simulink model "pendulum_cart"  (R2020a)
settings: Solver=VariableStepAuto  StartTime=0.0  StopTime=15.0  MaxStep=0.01  RelTol=1e-3
libraries: simulink x1, simulink_extras x1
settings Model: Creator=kiril_000  LastModifiedBy=kiril_000

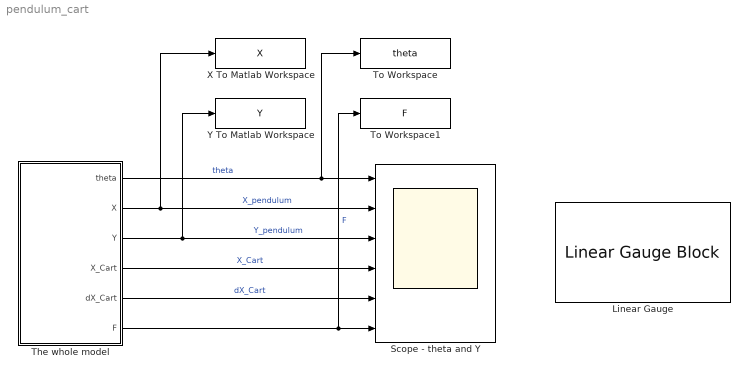
== system pendulum_cart ==
  Linear Gauge : LinearGaugeBlock  ScaleMin=-90  ScaleMax=90
  Scope - theta and Y : Scope  NumInputPorts=6
  The whole model : Subsystem  mask{m=1, M_Cart=3, l=1}
      mask prompts: m "Масса маятника"; M_Cart "Масса тележки"; l "Длина"
  To Workspace : ToWorkspace  VariableName=theta  SaveFormat=Timeseries  SampleTime=-1
  To Workspace1 : ToWorkspace  VariableName=F  SaveFormat=Timeseries  SampleTime=-1
  X To Matlab Workspace : ToWorkspace  VariableName=X  SampleTime=-1
      settings: Save2DSignal=2-D array (concatenate along first dimension)
  Y To Matlab Workspace : ToWorkspace  VariableName=Y  SampleTime=-1
      settings: Save2DSignal=2-D array (concatenate along first dimension)
  wires:
  The whole model/2(X) -> X To Matlab Workspace/1, Scope - theta and Y/2  "X_pendulum"
  The whole model/3(Y) -> Y To Matlab Workspace/1, Scope - theta and Y/3  "Y_pendulum"
  The whole model/1(theta) -> To Workspace/1, Scope - theta and Y/1  "theta"
  The whole model/4(X_Cart) -> Scope - theta and Y/4  "X_Cart"
  The whole model/5(dX_Cart) -> Scope - theta and Y/5  "dX_Cart"
  The whole model/6(F) -> To Workspace1/1, Scope - theta and Y/6  "F"

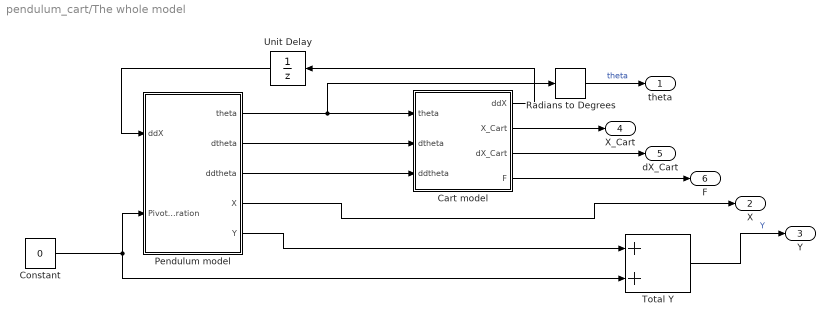
== system pendulum_cart/The whole model ==
  Cart model : Subsystem
  Constant : Constant  Value=0
  Pendulum model : Subsystem  mask{m=1, l=1, g=9.8, b=0.5}
      mask prompts: m "Масса"; l "Длина"; g "Ускорение свободного падения"; b "Коэффициент вязкости"
      mask init:
      | I = m * l^2;
  Radians to Degrees : simulink_extras/Transformations/Radians to Degrees
  Total Y : Sum
  Unit Delay : UnitDelay  SampleTime=-1  HasFrameUpgradeWarning=on
  theta : Outport
  X : Outport  Port=2
  Y : Outport  Port=3
  X_Cart : Outport  Port=4
  dX_Cart : Outport  Port=5
  F : Outport  Port=6
  wires:
  Radians to Degrees/1 -> theta/1  "theta"
  Cart model/1(ddX) -> Unit Delay/1
  Pendulum model/3(ddtheta) -> Cart model/3(ddtheta)
  Pendulum model/1(theta) -> Radians to Degrees/1, Cart model/1(theta)
  Pendulum model/5(Y) -> Total Y/1
  Pendulum model/4(X) -> X/1
  Pendulum model/2(dtheta) -> Cart model/2(dtheta)
  Total Y/1 -> Y/1  "Y"
  Constant/1 -> Total Y/2, Pendulum model/2(Pivot Acceleration)
  Cart model/2(X_Cart) -> X_Cart/1
  Cart model/3(dX_Cart) -> dX_Cart/1
  Cart model/4(F) -> F/1
  Unit Delay/1 -> Pendulum model/1(ddX)

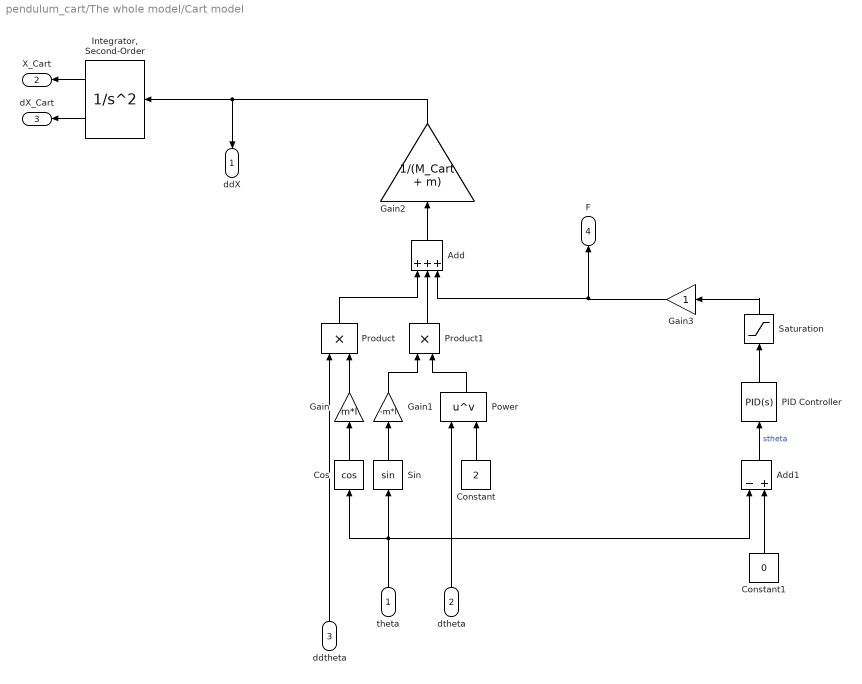
== system pendulum_cart/The whole model/Cart model ==
  theta : Inport
  dtheta : Inport  Port=2
  ddtheta : Inport  Port=3
  Add : Sum  Inputs=+++
  Add1 : Sum  Inputs=-+
  Constant : Constant  Value=2
  Constant1 : Constant  Value=0
  Cos : Trigonometry  Operator=cos
  Gain : Gain  Gain=m*l
  Gain1 : Gain  Gain=-m*l
  Gain2 : Gain  Gain=1/(M_Cart + m)
  Gain3 : Gain
  "Integrator, Second-Order" : SecondOrderIntegrator
  PID Controller : simulink/Continuous/PID Controller  Controller=PID  Form=Parallel  TimeDomain=Continuous-time  UseExternalTs=off  SampleTime=-1  IntegratorMethod=Forward Euler  FilterMethod=Forward Euler  ControllerParametersSource=internal  P=48  I=0  D=3  UseFilter=on  N=100  TunerSelectOption=Transfer Function Based (PID Tuner App)  InitialConditionSource=internal  InitialConditionForIntegrator=0  InitialConditionForFilter=0  DifferentiatorICPrevScaledInput=0  ExternalReset=none  TrackingMode=off  Kt=1  LimitOutput=off  UpperSaturationLimit=inf  LowerSaturationLimit=-inf  LinearizeAsGain=on  AntiWindupMode=none  Kb=1  POutMin=[]  POutMax=[]  IOutMin=[]  IOutMax=[]  DOutMin=[]  DOutMax=[]  NOutMin=[]  NOutMax=[]  SumOutMin=[]  SumOutMax=[]  SaturationOutMin=[]  SaturationOutMax=[]  PParamMin=[]  PParamMax=[]  IParamMin=[]  IParamMax=[]  DParamMin=[]  DParamMax=[]  NParamMin=[]  NParamMax=[]  KbParamMin=[]  KbParamMax=[]  KtParamMin=[]  KtParamMax=[]  KbOutMin=[]  KbOutMax=[]  KtOutMin=[]  KtOutMax=[]  IntegratorOutMin=[]  IntegratorOutMax=[]  FilterOutMin=[]  FilterOutMax=[]  SumI1OutMin=[]  SumI1OutMax=[]  SumI2OutMin=[]  SumI2OutMax=[]  SumI3OutMin=[]  SumI3OutMax=[]  SumI4OutMin=[]  SumI4OutMax=[]  SumDOutMin=[]  SumDOutMax=[]  DifferentiatorOutMin=[]  DifferentiatorOutMax=[]  FilterDiffOutCoefMin=[]  FilterDiffOutCoefMax=[]  ReciprocalOutMin=[]  ReciprocalOutMax=[]  SumDenOutMin=[]  SumDenOutMax=[]  SumNumOutMin=[]  SumNumOutMax=[]  DivideOutMin=[]  DivideOutMax=[]  UdiffTsProdOutMin=[]  UdiffTsProdOutMax=[]  NTsProdOutMin=[]  NTsProdOutMax=[]  UintegralTsProdOutMin=[]  UintegralTsProdOutMax=[]  UngainTsProdOutMin=[]  UngainTsProdOutMax=[]  IntegratorContinuousStateAttributes=''  IntegratorStateMustResolveToSignalObject=off  IntegratorRTWStateStorageClass=Auto  FilterContinuousStateAttributes=''  FilterStateMustResolveToSignalObject=off  FilterRTWStateStorageClass=Auto  ParallelPVariant=InternalParameters  IdealPVariant=Disabled  IVariant=InternalParameters  DVariant=InternalParameters  IntegratorVariant=Continuous  SatVariant=Disabled  AWVariant=Passthrough  PCopyVariant=Disabled  TRVariant=Disabled  FdbkBlocksVariant=Forward  IdealPFdbkVariant=Disabled  SatFdbkVariant=Disabled  DerivativeFilterVariant=ContFilter  NVariant=InternalParameters  NCopyVariant=Disabled  FilterICVariant=InternalICsFilter  IntegratorICVariant=InternalICs  ExternalResetVariant=Disabled  TRSumVariant=Passthrough  SumFdbkVariant=Disabled  SumVariant=Sum_PID  TsampFilterVariant=InternalTs  TsampNgainVariant=Passthrough  TsampIntegralVariant=Passthrough
  Power : Math  Operator=pow  SaturateOnIntegerOverflow=on
  Product : Product
  Product1 : Product
  Saturation : Saturate  UpperLimit=5  LowerLimit=-5
  Sin : Trigonometry
  ddX : Outport
  X_Cart : Outport  Port=2
  dX_Cart : Outport  Port=3
  F : Outport  Port=4
  wires:
  Sin/1 -> Gain1/1
  Cos/1 -> Gain/1
  Product1/1 -> Add/2
  Power/1 -> Product1/2
  Gain1/1 -> Product1/1
  Add/1 -> Gain2/1
  Constant/1 -> Power/2
  Gain/1 -> Product/2
  Product/1 -> Add/1
  dtheta/1 -> Power/1
  ddtheta/1 -> Product/1
  theta/1 -> Cos/1, Add1/1, Sin/1
  Gain2/1 -> ddX/1, "Integrator, Second-Order"/1
  "Integrator, Second-Order"/2 -> dX_Cart/1
  "Integrator, Second-Order"/1 -> X_Cart/1
  Constant1/1 -> Add1/2
  Add1/1 -> PID Controller/1  "stheta"
  PID Controller/1 -> Saturation/1
  Saturation/1 -> Gain3/1
  Gain3/1 -> F/1, Add/3

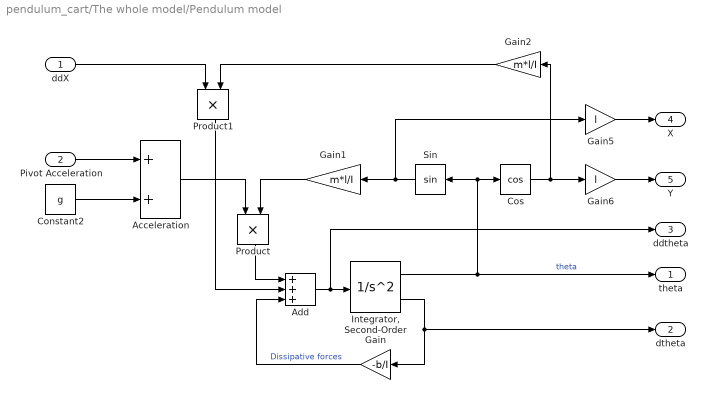
== system pendulum_cart/The whole model/Pendulum model ==
  ddX : Inport
  Pivot Acceleration : Inport  Port=2
  Acceleration : Sum
  Add : Sum  Inputs=+++
  Constant2 : Constant  Value=g
  Cos : Trigonometry  Operator=cos
  Gain : Gain  Gain=-b/I
  Gain1 : Gain  Gain=m*l/I
  Gain2 : Gain  Gain=m*l/I
  Gain5 : Gain  Gain=l
  Gain6 : Gain  Gain=l
  "Integrator, Second-Order" : SecondOrderIntegrator  ICX=deg2rad(5)
  Product : Product
  Product1 : Product
  Sin : Trigonometry
  theta : Outport
  dtheta : Outport  Port=2
  ddtheta : Outport  Port=3
  X : Outport  Port=4
  Y : Outport  Port=5
  wires:
  Sin/1 -> Gain1/1, Gain5/1
  "Integrator, Second-Order"/2 -> Gain/1, dtheta/1
  "Integrator, Second-Order"/1 -> Cos/1, Sin/1, theta/1  "theta"
  Gain1/1 -> Product/2
  Add/1 -> ddtheta/1, "Integrator, Second-Order"/1
  Gain/1 -> Add/3  "Dissipative forces"
  Cos/1 -> Gain6/1, Gain2/1
  Pivot Acceleration/1 -> Acceleration/1
  Constant2/1 -> Acceleration/2
  Acceleration/1 -> Product/1
  Product/1 -> Add/1
  Gain5/1 -> X/1
  Gain6/1 -> Y/1
  ddX/1 -> Product1/1
  Gain2/1 -> Product1/2
  Product1/1 -> Add/2
